simulink model "scenario2"  (R2018a)
settings: Solver=VariableStepAuto  StartTime=0.0  StopTime=35  RelTol=1e-3
undefined symbols (not defined in the file or in its folder): sigbuilder_block
libraries: fuzblock x1
settings Model: Creator=root  LastModifiedBy=root

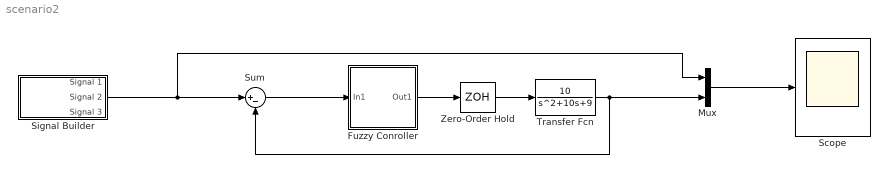
== system scenario2 ==
  Fuzzy Conroller : Subsystem
  Mux : Mux  Inputs=2
  Scope : Scope
  Signal Builder : Subsystem  Tag=STV Subsys  LoadFcn=sigbuilder_block('load');  StartFcn=sigbuilder_block('start');  StopFcn=sigbuilder_block('stop');  ClipboardFcn=sigbuilder_block('clipboard');  mask(Sigbuilder block){tuvar=[0:10]}
      mask help: Simulink:masks:SigbuilderBlock_MD
      mask init:
      | if ~strcmp(get_param(bdroot(gcbh),'SimulationStatus'),'stopped') tuvar = sigbuilder_block('maskInit'); end
      settings: CopyFcn=sigbuilder_block('copy');  DeleteFcn=sigbuilder_block('delete');  ModelCloseFcn=sigbuilder_block('modelClose');  PreSaveFcn=sigbuilder_block('preSave');  PauseFcn=sigbuilder_block('pause');  ContinueFcn=sigbuilder_block('continue');  NameChangeFcn=sigbuilder_block('namechange');  OpenFcn=sigbuilder_block('open',[433.5 83.25 558 417 ]);  CloseFcn=sigbuilder_block('close');
      mask Display: plot(0, 0, 100, 100,[2, 2, 32, 32, 2], [68, 8, 8, 68, 68],[32, 2], [38, 38], [32, 19, 2],[53, 60, 44], [32, 17, 17, 2],[16, 16, 31, 31]);txt = getActiveGroup(gcbh);text(2, 100, txt,'verticalAlignment', 'top');
  Sum : Sum  Inputs=|+-
  Transfer Fcn : TransferFcn  Numerator=[10]  Denominator=[1 10 9]
  Zero-Order Hold : ZeroOrderHold  SampleTime=0.01
  wires:
  Fuzzy Conroller/1(Out1) -> Zero-Order Hold/1
  Transfer Fcn/1 -> Mux/2, Sum/2
  Zero-Order Hold/1 -> Transfer Fcn/1
  Signal Builder/2(Signal 2) -> Mux/1, Sum/1
  Mux/1 -> Scope/1
  Sum/1 -> Fuzzy Conroller/1(In1)

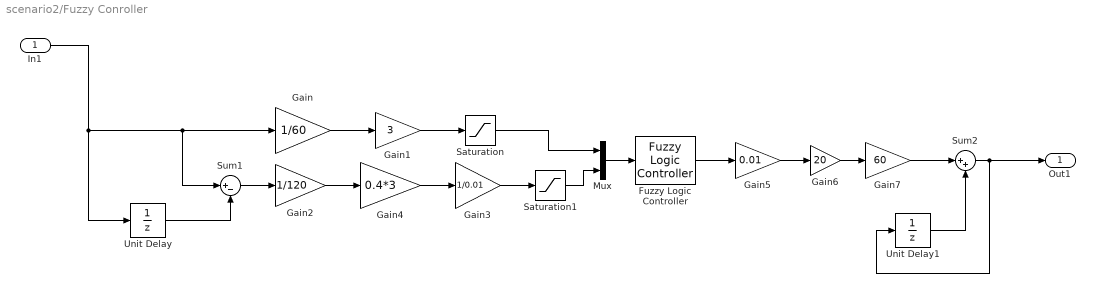
== system scenario2/Fuzzy Conroller ==
  In1 : Inport
  Fuzzy Logic Controller : fuzblock/Fuzzy Logic  Controller  FIS='satellite_8885'  OutputSampleNumber=101  DataType=single  FuzzifiedInputs=off  RuleFiringStrengths=off  RuleOutputs=off  AggregatedOutputs=off  SimulateUsing=Interpreted execution  OutOfRangeInputValueMessage=warning  NoRuleFiredMessage=warning  EmptyOutputFuzzySetMessage=warning
  Gain : Gain  Gain=1/60
  Gain1 : Gain  Gain=3
  Gain2 : Gain  Gain=1/120
  Gain3 : Gain  Gain=1/0.01
  Gain4 : Gain  Gain=0.4*3
  Gain5 : Gain  Gain=0.01
  Gain6 : Gain  Gain=20
  Gain7 : Gain  Gain=60
  Mux : Mux  Inputs=2
  Saturation : Saturate  UpperLimit=1  LowerLimit=-1
  Saturation1 : Saturate  UpperLimit=1  LowerLimit=-1
  Sum1 : Sum  Inputs=|+-
  Sum2 : Sum  Inputs=|++
  Unit Delay : UnitDelay  SampleTime=-1
  Unit Delay1 : UnitDelay  SampleTime=-1
  Out1 : Outport
  wires:
  Gain/1 -> Gain1/1
  Gain2/1 -> Gain4/1
  Saturation1/1 -> Mux/2
  In1/1 -> Unit Delay/1, Sum1/1, Gain/1
  Unit Delay/1 -> Sum1/2
  Sum2/1 -> Unit Delay1/1, Out1/1
  Saturation/1 -> Mux/1
  Unit Delay1/1 -> Sum2/2
  Gain4/1 -> Gain3/1
  Gain6/1 -> Gain7/1
  Gain7/1 -> Sum2/1
  Sum1/1 -> Gain2/1
  Gain1/1 -> Saturation/1
  Gain3/1 -> Saturation1/1
  Mux/1 -> Fuzzy Logic Controller/1
  Gain5/1 -> Gain6/1
  Fuzzy Logic Controller/1 -> Gain5/1

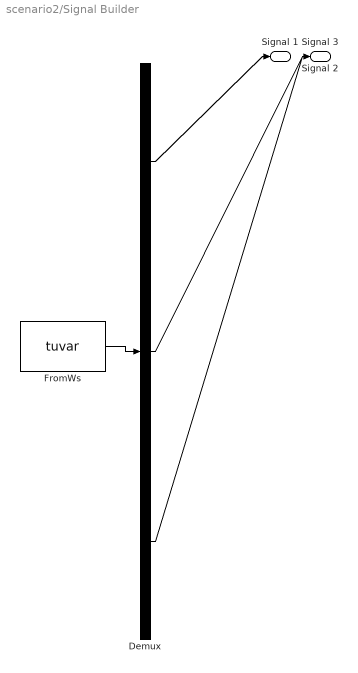
== system scenario2/Signal Builder ==
  Demux : Demux  Tag=STV Demux  Outputs=3
  FromWs : FromWorkspace  Tag=STV FromWs  VariableName=tuvar  SampleTime=0
      SigBuilderData=|
      | common.afterFinalStr = 'Extrapolate'
      | common.sampleTime = 0
      | dataSet.timeRange = [0 40]
      | dataSet.name = 'Group 1'
      | sbobj.Groups.Name = 'Group 1'
      | sbobj.Groups.Signals(1).Name = 'Signal 1'
      | sbobj.Groups.Signals(1).XData = [0 40]
      | sbobj.Groups.Signals(1).YData = [60 60]
      | sbobj.Groups.Signals(2).Name = 'Signal 2'
      | sbobj.Groups.Signals(2).XData = [0 4 4 8 8 40]
      | sbobj.Groups.Signals(2).YData = [60 60 20 20 40 40]
      | sbobj.Groups.Signals(3).Name = 'Signal 3'
      | sbobj.Groups.Signals(3).XData = [0 5 8 16 24 40]
      | sbobj.Groups.Signals(3).YData = [0.4 60 60 0.4 0.4 0.4]
      | sbobj.Groups.TimeRange = [0 40]
  Signal 1 : Outport  Tag=STV Outport
  Signal 2 : Outport  Tag=STV Outport  Port=2
  Signal 3 : Outport  Tag=STV Outport  Port=3
  wires:
  FromWs/1 -> Demux/1
  Demux/1 -> Signal 1/1
  Demux/2 -> Signal 2/1
  Demux/3 -> Signal 3/1
